simulink model "novamontagemrobo"  (R2018a)
settings: Solver=VariableStepAuto  StartTime=0.0  StopTime=120  RelTol=1e-3
model workspace: external: MATLAB File C:\Users\reigo\Downloads\robotica\DRIVE_ROBOTICA_NOSSO-20201226T192818Z-001\simulink\simulink\novamontagemrobo_DataFile.m (data not in the file)
values from neighbouring files (symbols this model uses):
  m = [207.61613 346.81729 366.65763 243.34094 10.76884 27.61521 3.40236]    [matlab.mat]
undefined symbols (not defined in the file or in its folder): smiData, X, Y, Z
libraries: sm_lib x58, nesl_utility x31
(part 3 of 3)

== matlab function novamontagemrobo/MATLAB Function5 ==
  data: posX output; posY output; parametro_robo input; valor_q_inv input; posZ output; tarefa input; qx output; qy output; qz output; caixa input
function [posX,posY,posZ,qx,qy,qz] = pos_caixa4(parametro_robo,valor_q_inv,tarefa,caixa)
coder.extrinsic('evalin')
qx=(pi/2);
qy=(pi/2)+pi/2;
qz=0;
xf=parametro_robo(7);
posX=0;
posY=3.4-xf;
posZ=0.9076;

if caixa>=2 && caixa<4
    posX=0;
    posY=3.1-xf;
    posZ=0.90764;
end

if caixa>=4 && caixa <6
    posX=0;
    posY=2.8-xf;
    posZ=0.90764;
end

if caixa==6
    posX=0;
    posY=2.5-xf;
    posZ=0.90764;
end


if caixa>7
    posX=0.80015;
    posY=-2.04985+xf;
    posZ= 0.58564;
    qy=0;
end

if caixa==7
qx=tarefa(4)+(pi/2);
qy=tarefa(6)+(pi/2);
qz=-tarefa(5);
L1=parametro_robo(1);L2=parametro_robo(2); L3=parametro_robo(3);L4=parametro_robo(4);
E1=parametro_robo(5);E2=parametro_robo(6);yf=parametro_robo(8);
zf=parametro_robo(9);


q1=valor_q_inv(1);q2=valor_q_inv(2);q3=valor_q_inv(3);q4=valor_q_inv(4);
q5=valor_q_inv(5);q6=valor_q_inv(6);


 R1_0 = [cos(q1) -sin(q1) 0 0; sin(q1) cos(q1) 0 0; 0 0 1 0; 0 0 0 1];
 D1_0 = [1 0 0 E1; 0 1 0 0; 0 0 1 L1; 0 0 0 1];
 T1_0 = R1_0*D1_0;
 R2_1 = [cos(q2) 0 sin(q2) 0; 0 1 0 0; -sin(q2) 0 cos(q2) 0; 0 0 0 1];
 D2_1 = [1 0 0 L2; 0 1 0 0; 0 0 1 0; 0 0 0 1];
 T2_1 = R2_1*D2_1;
 T2_0 = T1_0*T2_1;
 R3_2 = [cos(q3) 0 sin(q3) 0; 0 1 0 0; -sin(q3) 0 cos(q3) 0; 0 0 0 1];
 D3_2 = [1 0 0 L3; 0 1 0 0; 0 0 1 E2; 0 0 0 1];
 T3_2 = R3_2*D3_2;
 T3_0 = T2_0*T3_2;
 R4_3 = [1 0 0 0; 0 cos(q4) -sin(q4) 0; 0 sin(q4) cos(q4) 0; 0 0 0 1];
 T4_3 = R4_3;
 T4_0 =T3_0*T4_3;
 R5_4 = [cos(q5) 0 sin(q5) 0; 0 1 0 0; -sin(q5) 0 cos(q5) 0; 0 0 0 1];
 T5_4 = R5_4;
 T5_0 = T4_0*T5_4;                               
 R6_5 = [1 0 0 0; 0 cos(q6) -sin(q6) 0; 0 sin(q6) cos(q6) 0; 0 0 0 1];
 T6_5 = R6_5;
 T6_0 = T5_0*T6_5; 
 D7_6 = [1 0 0 L4; 0 1 0 yf; 0 0 1 zf; 0 0 0 1];
 T7_6 = D7_6;
 T7_0=T6_0*T7_6;
 pos=T7_0(1:3,4);
posX=pos(1);
posY=pos(2);
posZ=pos(3);
end
end

== matlab function novamontagemrobo/MATLAB Function6 ==
  data: posX output; posY output; parametro_robo input; valor_q_inv input; posZ output; tarefa input; qx output; qy output; qz output; caixa input
function [posX,posY,posZ,qx,qy,qz] = pos_caixa2(parametro_robo,valor_q_inv,tarefa,caixa)
coder.extrinsic('evalin')
qx=(pi/2);
qy=(pi/2)+pi/2;
qz=0;
xf=parametro_robo(7);
posX=0;
posY=2.8-xf;
posZ=0.90764;

if caixa==2
    posX=0;
    posY=2.5-xf;
    posZ=0.90764;
end

if caixa>3
    posX=0.80015;
    posY=-2.04985+xf;
    posZ=0.24564;
    qy=0;
end

if caixa==3
qx=tarefa(4)+(pi/2);
qy=tarefa(6)+(pi/2);
qz=-tarefa(5);
L1=parametro_robo(1);L2=parametro_robo(2); L3=parametro_robo(3);L4=parametro_robo(4);
E1=parametro_robo(5);E2=parametro_robo(6);yf=parametro_robo(8);
zf=parametro_robo(9);


q1=valor_q_inv(1);q2=valor_q_inv(2);q3=valor_q_inv(3);q4=valor_q_inv(4);
q5=valor_q_inv(5);q6=valor_q_inv(6);


 R1_0 = [cos(q1) -sin(q1) 0 0; sin(q1) cos(q1) 0 0; 0 0 1 0; 0 0 0 1];
 D1_0 = [1 0 0 E1; 0 1 0 0; 0 0 1 L1; 0 0 0 1];
 T1_0 = R1_0*D1_0;
 R2_1 = [cos(q2) 0 sin(q2) 0; 0 1 0 0; -sin(q2) 0 cos(q2) 0; 0 0 0 1];
 D2_1 = [1 0 0 L2; 0 1 0 0; 0 0 1 0; 0 0 0 1];
 T2_1 = R2_1*D2_1;
 T2_0 = T1_0*T2_1;
 R3_2 = [cos(q3) 0 sin(q3) 0; 0 1 0 0; -sin(q3) 0 cos(q3) 0; 0 0 0 1];
 D3_2 = [1 0 0 L3; 0 1 0 0; 0 0 1 E2; 0 0 0 1];
 T3_2 = R3_2*D3_2;
 T3_0 = T2_0*T3_2;
 R4_3 = [1 0 0 0; 0 cos(q4) -sin(q4) 0; 0 sin(q4) cos(q4) 0; 0 0 0 1];
 T4_3 = R4_3;
 T4_0 =T3_0*T4_3;
 R5_4 = [cos(q5) 0 sin(q5) 0; 0 1 0 0; -sin(q5) 0 cos(q5) 0; 0 0 0 1];
 T5_4 = R5_4;
 T5_0 = T4_0*T5_4;                               
 R6_5 = [1 0 0 0; 0 cos(q6) -sin(q6) 0; 0 sin(q6) cos(q6) 0; 0 0 0 1];
 T6_5 = R6_5;
 T6_0 = T5_0*T6_5; 
 D7_6 = [1 0 0 L4; 0 1 0 yf; 0 0 1 zf; 0 0 0 1];
 T7_6 = D7_6;
 T7_0=T6_0*T7_6;
 pos=T7_0(1:3,4);
posX=pos(1);
posY=pos(2);
posZ=pos(3);
end
end
